simulink model "tora"  (Simulink 6.6)
settings: Solver=ode23t  StartTime=0.0  StopTime=50  RelTol=1e-3
undefined symbols (not defined in the file or in its folder): tora_control
settings Model: Creator=nsz  LastModifiedBy=nsz  ExtModeTrigMode=oneshot  ExtModeArmWhenConnect=off  ExtModeAutoUpdateStatusClock=off
settings DataIOCC: LimitDataPoints=off  SaveOutput=off  SaveTime=off
settings OptimizationCC: BooleanDataType=off
settings DebuggingCC: SignalResolutionControl=TryResolveAllWithWarning  SolverPrmCheckMsg=none  MultiTaskDSMMsg=warning  MultiTaskCondExecSysMsg=none  StrictBusMsg=None
settings HardwareCC: TargetUnknown=on
settings RTWCC: IncludeERTFirstTime=on
settings GRTTargetCC: ModelReferenceCompliant=off  MatFileLogging=off

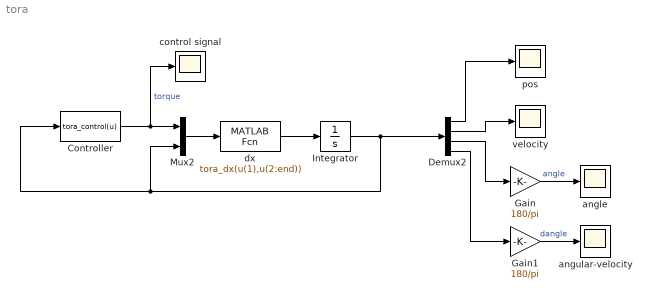
== system tora ==
  Controller : MATLABFcn  MATLABFcn=tora_control(u)  OutputDimensions=1
  Demux2 : Demux
  Gain : Gain  Gain=180/pi
  Gain1 : Gain  Gain=180/pi
  Integrator : Integrator  InitialCondition=[0.1; 0; 60/180*pi; 0]
  Mux2 : Mux  Inputs=2
  angle : Scope
      settings: YMin=-0.45  YMax=0.55
  angular-velocity : Scope
      settings: YMin=-0.045  YMax=0.055
  control signal : Scope
      settings: YMin=-0.2  YMax=0.175
  dx : MATLABFcn  MATLABFcn=tora_dx(u(1),u(2:end))  OutputDimensions=4
  pos : Scope
      settings: YMin=-0.1  YMax=0.11
  velocity : Scope
      settings: YMin=-0.0009  YMax=0.0009
  wires:
  Mux2/1 -> dx/1
  dx/1 -> Integrator/1
  Controller/1 -> control signal/1, Mux2/1  "torque"
  Demux2/1 -> pos/1
  Demux2/2 -> velocity/1
  Integrator/1 -> Demux2/1, Mux2/2, Controller/1
  Gain1/1 -> angular-velocity/1  "dangle"
  Demux2/4 -> Gain1/1
  Demux2/3 -> Gain/1
  Gain/1 -> angle/1  "angle"
